simulink model "inner_loop_controller"  (R2019b)
settings: Solver=VariableStepAuto  StartTime=0.0  StopTime=10.0  RelTol=1e-3
settings Model: Creator=wangcanye  LastModifiedBy=wangcanye

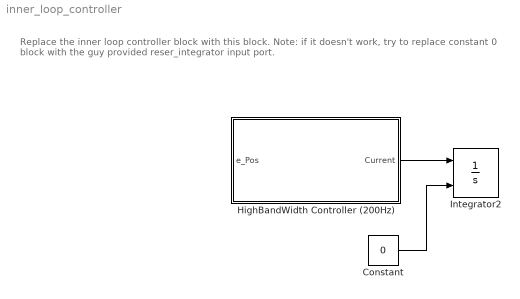
== system inner_loop_controller ==
  note: Replace the inner loop controller block with this block.
      |
      | Note: if it doesn't work, try to replace constant 0 block with the guy provided reser_integrator input port.
  Constant : Constant  Value=0
  HighBandWidth Controller (200Hz) : Subsystem
  Integrator2 : Integrator  ExternalReset=rising  LimitOutput=on  UpperSaturationLimit=3  LowerSaturationLimit=-3
  wires:
  HighBandWidth Controller (200Hz)/1(Current) -> Integrator2/1
  Constant/1 -> Integrator2/2

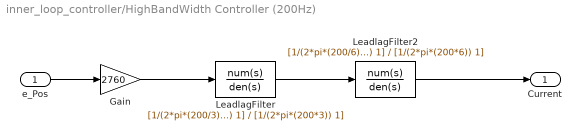
== system inner_loop_controller/HighBandWidth Controller (200Hz) ==
  e_Pos : Inport
  Gain : Gain  Gain=2760
  LeadlagFilter : TransferFcn  Numerator=[1/(2*pi*(200/3)) 1]  Denominator=[1/(2*pi*(200*3)) 1]
  LeadlagFilter2 : TransferFcn  Numerator=[1/(2*pi*(200/6)) 1]  Denominator=[1/(2*pi*(200*6)) 1]
  Current : Outport
  wires:
  Gain/1 -> LeadlagFilter/1
  e_Pos/1 -> Gain/1
  LeadlagFilter/1 -> LeadlagFilter2/1
  LeadlagFilter2/1 -> Current/1
